simulink model "N3Z_tonetestprevious"  (R2014b)
settings: Solver=ode3  SolverMode=SingleTasking  StartTime=0.0  StopTime=1e-4  FixedStep=fpgaclk  RelTol=1e-3
PreLoadFcn:
  | %fpgaclk=1/32.768e6
  | fpgaclk=1/49.162e6
  | 
  | SerialData=[1,zeros(1,11),1,0,0,1]
  | load ../N3workingG/window
  | win=win';  %Go back to using flatter and wider windowed sync function
  | %load ../N3workingG/hanning    %use Hahn window
  | 
  | load ../N3workingG/PREemphasis   %For pre-empasis and deemphasis FIRs
  | 
  | %LUT3=xls2LUT2('../IQI_Qdemod.xls'); LUT3
  | load ../N3workingG/LUT3
  | load ../N3workingG/FIRiq2
  | % xls2LUT
  | 
  | GetProgFiles
  | 
  | PinAssignments    %Get Pin references for TE0722
  | 
  | 
  | 
  | 
  | 
  | %LCD
  | LCDdata=[LCD_D7,LCD_D6,LCD_D5,LCD_D4,LCD_D3,LCD_D2,LCD_D1,LCD_D0] %Note MSB...LSB!
  | LCDctrl=[LCD_E,LCD_RW,LCD_RS];
  | 
  | %for RS232 on pins 3 and 5 of USBB
  | 
  | %BT chip connections for WT12
  | 
  | RX_BT=RXD
  | TX_BT=TXD
  | 
  | RST_BB=RES
  | 
  | %PCMC=PCMC
  | %PCMS=PCMS
  | %PCMI=PCMI
  | %PCMO=PCMO
  | 
  | %Aliases:
  | SRDBT=PCMI
  | STDBT=PCMO
  | SCLK_BT=PCMC
  | SFS_BT=PCMS
  | 
  | %ADC control
  | 
  | %SDOA=SDOA
  | %SDOB=SDOB
  | %SCK=SCK
  | CONV=Csbar
  | CAL=Cal
  | 
  | ADC_G=[ADC_G3,ADC_G2,ADC_G1,ADC_G0]
  | %PD settings hard coded now
  | 
  | %%%%%%
  | TX_LOW=TX_Low
  | ... (+11 lines)
StartFcn:
  | SerialData=[1,zeros(1,11),1,0,0,1]
values from neighbouring files (symbols this model uses):
  ADC_G0 = {'P10'}    [PinAssignments.m]
  ADC_G1 = {'P11'}    [PinAssignments.m]
  ADC_G2 = {'N14'}    [PinAssignments.m]
  ADC_G3 = {'M11'}    [PinAssignments.m]
  Cal = {'L12'}    [PinAssignments.m]
  Csbar = {'M12'}    [PinAssignments.m]
  LCD_D0 = {'J13'}    [PinAssignments.m]
  LCD_D1 = {'J14'}    [PinAssignments.m]
  LCD_D2 = {'F15'}    [PinAssignments.m]
  LCD_D3 = {'H14'}    [PinAssignments.m]
  LCD_D4 = {'G12'}    [PinAssignments.m]
  LCD_D5 = {'L15'}    [PinAssignments.m]
  LCD_D6 = {'M14'}    [PinAssignments.m]
  LCD_D7 = {'K15'}    [PinAssignments.m]
  PCMC = {'H11'}    [PinAssignments.m]
  PCMI = {'H12'}    [PinAssignments.m]
  PCMO = {'N13'}    [PinAssignments.m]
  PCMS = {'M10'}    [PinAssignments.m]
  RES = {'G11'}    [PinAssignments.m]
  RXD = {'H13'}    [PinAssignments.m]
  TX_Low = {'P15'}    [PinAssignments.m]
  TXD = {'P13'}    [PinAssignments.m]
undefined symbols (not defined in the file or in its folder): AXI4, FIRRX, FIRTX, Lite
libraries: xbsIndex_r4 x1250, MyFunctions x43
(part 9 of 10)

== system N3Z_tonetestprevious/ToneDetect/OutputRegister/Subsystem4 ==
  Data : Inport
  PortId : Inport  Port=2
  Write : Inport  Port=3
  Logical : xbsIndex_r4/Logical  logical_function=AND  inputs=2  en=off  latency=0  precision=Full  arith_type=Unsigned  n_bits=8  bin_pt=2  align_bp=on  dbl_ovrd=off  block_type=logical
      settings: xl_area=[1 0 0 1 0 0 0]  block_version=VER_STRING_GOES_HERE
  PortAddress : xbsIndex_r4/Constant  const=2  gui_display_data_type=Fixed-point  arith_type=Unsigned  n_bits=8  bin_pt=0  preci_type=Single  exp_width=8  frac_width=24  explicit_period=on  period=fpgaclk  equ=P=C  opselect=C  inp2=PCIN>>17  opr=+  inp1=P  carry=CIN  dbl_ovrd=off  block_type=constant
      settings: block_version=VER_STRING_GOES_HERE
  Register1 : xbsIndex_r4/Register  init=0  rst=off  en=on  dbl_ovrd=off  block_type=register
      settings: xl_area=[4 8 0 0 0 0 0]  block_version=VER_STRING_GOES_HERE
  Relational1 : xbsIndex_r4/Relational  mode=a=b  op_type=Bool  en=off  latency=0  dbl_ovrd=off  block_type=relational
      settings: xl_area=[2 0 0 4 0 0 0]  block_version=VER_STRING_GOES_HERE
  LatchedData : Outport
  wires:
  Relational1/1 -> Logical/1
  Logical/1 -> Register1/2
  PortAddress/1 -> Relational1/2
  Data/1 -> Register1/1
  PortId/1 -> Relational1/1
  Write/1 -> Logical/2
  Register1/1 -> LatchedData/1

== system N3Z_tonetestprevious/ToneDetect/OutputRegister/Subsystem5 ==
  Data : Inport
  PortId : Inport  Port=2
  Write : Inport  Port=3
  Logical : xbsIndex_r4/Logical  logical_function=AND  inputs=2  en=off  latency=0  precision=Full  arith_type=Unsigned  n_bits=8  bin_pt=2  align_bp=on  dbl_ovrd=off  block_type=logical
      settings: xl_area=[1 0 0 1 0 0 0]  block_version=VER_STRING_GOES_HERE
  PortAddress : xbsIndex_r4/Constant  const=8  gui_display_data_type=Fixed-point  arith_type=Unsigned  n_bits=8  bin_pt=0  preci_type=Single  exp_width=8  frac_width=24  explicit_period=on  period=fpgaclk  equ=P=C  opselect=C  inp2=PCIN>>17  opr=+  inp1=P  carry=CIN  dbl_ovrd=off  block_type=constant
      settings: block_version=VER_STRING_GOES_HERE
  Register1 : xbsIndex_r4/Register  init=0  rst=off  en=on  dbl_ovrd=off  block_type=register
      settings: xl_area=[4 8 0 0 0 0 0]  block_version=VER_STRING_GOES_HERE
  Relational1 : xbsIndex_r4/Relational  mode=a=b  op_type=Bool  en=off  latency=0  dbl_ovrd=off  block_type=relational
      settings: xl_area=[2 0 0 4 0 0 0]  block_version=VER_STRING_GOES_HERE
  LatchedData : Outport
  Strobe : Outport  Port=2
  wires:
  Relational1/1 -> Logical/1
  Logical/1 -> Register1/2, Strobe/1
  PortAddress/1 -> Relational1/2
  Data/1 -> Register1/1
  PortId/1 -> Relational1/1
  Write/1 -> Logical/2
  Register1/1 -> LatchedData/1

== system N3Z_tonetestprevious/ToneDetect/OutputRegister/Subsystem6 ==
  Data : Inport
  PortId : Inport  Port=2
  Write : Inport  Port=3
  Logical : xbsIndex_r4/Logical  logical_function=AND  inputs=2  en=off  latency=0  precision=Full  arith_type=Unsigned  n_bits=8  bin_pt=2  align_bp=on  dbl_ovrd=off  block_type=logical
      settings: xl_area=[1 0 0 1 0 0 0]  block_version=VER_STRING_GOES_HERE
  PortAddress : xbsIndex_r4/Constant  const=13  gui_display_data_type=Fixed-point  arith_type=Unsigned  n_bits=8  bin_pt=0  preci_type=Single  exp_width=8  frac_width=24  explicit_period=on  period=fpgaclk  equ=P=C  opselect=C  inp2=PCIN>>17  opr=+  inp1=P  carry=CIN  dbl_ovrd=off  block_type=constant
      settings: block_version=VER_STRING_GOES_HERE
  Register1 : xbsIndex_r4/Register  init=0  rst=off  en=on  dbl_ovrd=off  block_type=register
      settings: xl_area=[4 8 0 0 0 0 0]  block_version=VER_STRING_GOES_HERE
  Relational1 : xbsIndex_r4/Relational  mode=a=b  op_type=Bool  en=off  latency=0  dbl_ovrd=off  block_type=relational
      settings: xl_area=[2 0 0 4 0 0 0]  block_version=VER_STRING_GOES_HERE
  LatchedData : Outport
  Strobe : Outport  Port=2
  wires:
  Relational1/1 -> Logical/1
  Logical/1 -> Register1/2, Strobe/1
  PortAddress/1 -> Relational1/2
  Data/1 -> Register1/1
  PortId/1 -> Relational1/1
  Write/1 -> Logical/2
  Register1/1 -> LatchedData/1

== system N3Z_tonetestprevious/ToneDetect/OutputRegister/Subsystem7 ==
  Data : Inport
  PortId : Inport  Port=2
  Write : Inport  Port=3
  Logical : xbsIndex_r4/Logical  logical_function=AND  inputs=2  en=off  latency=0  precision=Full  arith_type=Unsigned  n_bits=8  bin_pt=2  align_bp=on  dbl_ovrd=off  block_type=logical
      settings: xl_area=[1 0 0 1 0 0 0]  block_version=VER_STRING_GOES_HERE
  PortAddress : xbsIndex_r4/Constant  const=18  gui_display_data_type=Fixed-point  arith_type=Unsigned  n_bits=8  bin_pt=0  preci_type=Single  exp_width=8  frac_width=24  explicit_period=on  period=fpgaclk  equ=P=C  opselect=C  inp2=PCIN>>17  opr=+  inp1=P  carry=CIN  dbl_ovrd=off  block_type=constant
      settings: block_version=VER_STRING_GOES_HERE
  Register1 : xbsIndex_r4/Register  init=0  rst=off  en=on  dbl_ovrd=off  block_type=register
      settings: xl_area=[4 8 0 0 0 0 0]  block_version=VER_STRING_GOES_HERE
  Relational1 : xbsIndex_r4/Relational  mode=a=b  op_type=Bool  en=off  latency=0  dbl_ovrd=off  block_type=relational
      settings: xl_area=[2 0 0 4 0 0 0]  block_version=VER_STRING_GOES_HERE
  LatchedData : Outport
  Strobe : Outport  Port=2
  wires:
  Relational1/1 -> Logical/1
  Logical/1 -> Register1/2, Strobe/1
  PortAddress/1 -> Relational1/2
  Data/1 -> Register1/1
  PortId/1 -> Relational1/1
  Write/1 -> Logical/2
  Register1/1 -> LatchedData/1

== system N3Z_tonetestprevious/ToneDetect/OutputRegister/Subsystem8 ==
  Data : Inport
  PortId : Inport  Port=2
  Write : Inport  Port=3
  Logical : xbsIndex_r4/Logical  logical_function=AND  inputs=2  en=off  latency=0  precision=Full  arith_type=Unsigned  n_bits=8  bin_pt=2  align_bp=on  dbl_ovrd=off  block_type=logical
      settings: xl_area=[1 0 0 1 0 0 0]  block_version=VER_STRING_GOES_HERE
  PortAddress : xbsIndex_r4/Constant  const=23  gui_display_data_type=Fixed-point  arith_type=Unsigned  n_bits=8  bin_pt=0  preci_type=Single  exp_width=8  frac_width=24  explicit_period=on  period=fpgaclk  equ=P=C  opselect=C  inp2=PCIN>>17  opr=+  inp1=P  carry=CIN  dbl_ovrd=off  block_type=constant
      settings: block_version=VER_STRING_GOES_HERE
  Register1 : xbsIndex_r4/Register  init=0  rst=off  en=on  dbl_ovrd=off  block_type=register
      settings: xl_area=[4 8 0 0 0 0 0]  block_version=VER_STRING_GOES_HERE
  Relational1 : xbsIndex_r4/Relational  mode=a=b  op_type=Bool  en=off  latency=0  dbl_ovrd=off  block_type=relational
      settings: xl_area=[2 0 0 4 0 0 0]  block_version=VER_STRING_GOES_HERE
  LatchedData : Outport
  Strobe : Outport  Port=2
  wires:
  Relational1/1 -> Logical/1
  Logical/1 -> Register1/2, Strobe/1
  PortAddress/1 -> Relational1/2
  Data/1 -> Register1/1
  PortId/1 -> Relational1/1
  Write/1 -> Logical/2
  Register1/1 -> LatchedData/1

== system N3Z_tonetestprevious/ToneDetect/OutputRegister/Subsystem9 ==
  Data : Inport
  PortId : Inport  Port=2
  Write : Inport  Port=3
  Logical : xbsIndex_r4/Logical  logical_function=AND  inputs=2  en=off  latency=0  precision=Full  arith_type=Unsigned  n_bits=8  bin_pt=2  align_bp=on  dbl_ovrd=off  block_type=logical
      settings: xl_area=[1 0 0 1 0 0 0]  block_version=VER_STRING_GOES_HERE
  PortAddress : xbsIndex_r4/Constant  const=9  gui_display_data_type=Fixed-point  arith_type=Unsigned  n_bits=8  bin_pt=0  preci_type=Single  exp_width=8  frac_width=24  explicit_period=on  period=fpgaclk  equ=P=C  opselect=C  inp2=PCIN>>17  opr=+  inp1=P  carry=CIN  dbl_ovrd=off  block_type=constant
      settings: block_version=VER_STRING_GOES_HERE
  Register1 : xbsIndex_r4/Register  init=0  rst=off  en=on  dbl_ovrd=off  block_type=register
      settings: xl_area=[4 8 0 0 0 0 0]  block_version=VER_STRING_GOES_HERE
  Relational1 : xbsIndex_r4/Relational  mode=a=b  op_type=Bool  en=off  latency=0  dbl_ovrd=off  block_type=relational
      settings: xl_area=[2 0 0 4 0 0 0]  block_version=VER_STRING_GOES_HERE
  LatchedData : Outport
  Strobe : Outport  Port=2
  wires:
  Relational1/1 -> Logical/1
  Logical/1 -> Register1/2, Strobe/1
  PortAddress/1 -> Relational1/2
  Data/1 -> Register1/1
  PortId/1 -> Relational1/1
  Write/1 -> Logical/2
  Register1/1 -> LatchedData/1

== system N3Z_tonetestprevious/User_Interface/OutputRegister/Subsystem ==
  Data : Inport
  PortId : Inport  Port=2
  Write : Inport  Port=3
  Logical : xbsIndex_r4/Logical  logical_function=AND  inputs=2  en=off  latency=0  precision=Full  arith_type=Unsigned  n_bits=8  bin_pt=2  align_bp=on  dbl_ovrd=off  block_type=logical
      settings: xl_area=[1 0 0 1 0 0 0]  block_version=VER_STRING_GOES_HERE
  PortAddress : xbsIndex_r4/Constant  const=0  gui_display_data_type=Fixed-point  arith_type=Unsigned  n_bits=8  bin_pt=0  preci_type=Single  exp_width=8  frac_width=24  explicit_period=on  period=fpgaclk  equ=P=C  opselect=C  inp2=PCIN>>17  opr=+  inp1=P  carry=CIN  dbl_ovrd=off  block_type=constant
      settings: block_version=VER_STRING_GOES_HERE
  Register1 : xbsIndex_r4/Register  init=0  rst=off  en=on  dbl_ovrd=off  block_type=register
      settings: xl_area=[4 8 0 0 0 0 0]  block_version=VER_STRING_GOES_HERE
  Relational1 : xbsIndex_r4/Relational  mode=a=b  op_type=Bool  en=off  latency=0  dbl_ovrd=off  block_type=relational
      settings: xl_area=[2 0 0 4 0 0 0]  block_version=VER_STRING_GOES_HERE
  LatchedData : Outport
  Strobe : Outport  Port=2
  wires:
  Relational1/1 -> Logical/1
  Logical/1 -> Register1/2, Strobe/1
  PortAddress/1 -> Relational1/2
  Data/1 -> Register1/1
  PortId/1 -> Relational1/1
  Write/1 -> Logical/2
  Register1/1 -> LatchedData/1

== system N3Z_tonetestprevious/User_Interface/OutputRegister/Subsystem1 ==
  Data : Inport
  PortId : Inport  Port=2
  Write : Inport  Port=3
  Logical : xbsIndex_r4/Logical  logical_function=AND  inputs=2  en=off  latency=0  precision=Full  arith_type=Unsigned  n_bits=8  bin_pt=2  align_bp=on  dbl_ovrd=off  block_type=logical
      settings: xl_area=[1 0 0 1 0 0 0]  block_version=VER_STRING_GOES_HERE
  PortAddress : xbsIndex_r4/Constant  const=1  gui_display_data_type=Fixed-point  arith_type=Unsigned  n_bits=8  bin_pt=0  preci_type=Single  exp_width=8  frac_width=24  explicit_period=on  period=fpgaclk  equ=P=C  opselect=C  inp2=PCIN>>17  opr=+  inp1=P  carry=CIN  dbl_ovrd=off  block_type=constant
      settings: block_version=VER_STRING_GOES_HERE
  Register1 : xbsIndex_r4/Register  init=0  rst=off  en=on  dbl_ovrd=off  block_type=register
      settings: xl_area=[4 8 0 0 0 0 0]  block_version=VER_STRING_GOES_HERE
  Register2 : xbsIndex_r4/Register  init=0  rst=off  en=off  dbl_ovrd=off  block_type=register
      settings: xl_area=[1 1 0 0 0 0 0]  block_version=VER_STRING_GOES_HERE
  Register3 : xbsIndex_r4/Register  init=0  rst=off  en=off  dbl_ovrd=off  block_type=register
      settings: xl_area=[1 1 0 0 0 0 0]  block_version=VER_STRING_GOES_HERE
  Relational1 : xbsIndex_r4/Relational  mode=a=b  op_type=Bool  en=off  latency=0  dbl_ovrd=off  block_type=relational
      settings: xl_area=[2 0 0 4 0 0 0]  block_version=VER_STRING_GOES_HERE
  pulse2 : Subsystem
  LatchedData : Outport
  MemWrite : Outport  Port=2
  wires:
  Relational1/1 -> Logical/1
  Logical/1 -> Register1/2, Register3/1
  PortAddress/1 -> Relational1/2
  Data/1 -> Register1/1
  PortId/1 -> Relational1/1
  Write/1 -> Logical/2
  Register1/1 -> LatchedData/1
  Register2/1 -> pulse2/1(In1)
  Register3/1 -> Register2/1
  pulse2/1(Out1) -> MemWrite/1

== system N3Z_tonetestprevious/User_Interface/OutputRegister/Subsystem10 ==
  Data : Inport
  PortId : Inport  Port=2
  Write : Inport  Port=3
  Logical : xbsIndex_r4/Logical  logical_function=AND  inputs=2  en=off  latency=0  precision=Full  arith_type=Unsigned  n_bits=8  bin_pt=2  align_bp=on  dbl_ovrd=off  block_type=logical
      settings: xl_area=[1 0 0 1 0 0 0]  block_version=VER_STRING_GOES_HERE
  PortAddress : xbsIndex_r4/Constant  const=10  gui_display_data_type=Fixed-point  arith_type=Unsigned  n_bits=8  bin_pt=0  preci_type=Single  exp_width=8  frac_width=24  explicit_period=on  period=fpgaclk  equ=P=C  opselect=C  inp2=PCIN>>17  opr=+  inp1=P  carry=CIN  dbl_ovrd=off  block_type=constant
      settings: block_version=VER_STRING_GOES_HERE
  Register1 : xbsIndex_r4/Register  init=floor(30022/256)  rst=off  en=on  dbl_ovrd=off  block_type=register
      settings: xl_area=[4 8 0 0 0 0 0]  block_version=VER_STRING_GOES_HERE
  Relational1 : xbsIndex_r4/Relational  mode=a=b  op_type=Bool  en=off  latency=0  dbl_ovrd=off  block_type=relational
      settings: xl_area=[2 0 0 4 0 0 0]  block_version=VER_STRING_GOES_HERE
  LatchedData : Outport
  wires:
  Relational1/1 -> Logical/1
  Logical/1 -> Register1/2
  PortAddress/1 -> Relational1/2
  Data/1 -> Register1/1
  PortId/1 -> Relational1/1
  Write/1 -> Logical/2
  Register1/1 -> LatchedData/1

== system N3Z_tonetestprevious/User_Interface/OutputRegister/Subsystem11 ==
  Data : Inport
  PortId : Inport  Port=2
  Write : Inport  Port=3
  Logical : xbsIndex_r4/Logical  logical_function=AND  inputs=2  en=off  latency=0  precision=Full  arith_type=Unsigned  n_bits=8  bin_pt=2  align_bp=on  dbl_ovrd=off  block_type=logical
      settings: xl_area=[1 0 0 1 0 0 0]  block_version=VER_STRING_GOES_HERE
  PortAddress : xbsIndex_r4/Constant  const=11  gui_display_data_type=Fixed-point  arith_type=Unsigned  n_bits=8  bin_pt=0  preci_type=Single  exp_width=8  frac_width=24  explicit_period=on  period=fpgaclk  equ=P=C  opselect=C  inp2=PCIN>>17  opr=+  inp1=P  carry=CIN  dbl_ovrd=off  block_type=constant
      settings: block_version=VER_STRING_GOES_HERE
  Register1 : xbsIndex_r4/Register  init=mod(30022 ,256)  rst=off  en=on  dbl_ovrd=off  block_type=register
      settings: xl_area=[4 8 0 0 0 0 0]  block_version=VER_STRING_GOES_HERE
  Relational1 : xbsIndex_r4/Relational  mode=a=b  op_type=Bool  en=off  latency=0  dbl_ovrd=off  block_type=relational
      settings: xl_area=[2 0 0 4 0 0 0]  block_version=VER_STRING_GOES_HERE
  LatchedData : Outport
  wires:
  Relational1/1 -> Logical/1
  Logical/1 -> Register1/2
  PortAddress/1 -> Relational1/2
  Data/1 -> Register1/1
  PortId/1 -> Relational1/1
  Write/1 -> Logical/2
  Register1/1 -> LatchedData/1

== system N3Z_tonetestprevious/User_Interface/OutputRegister/Subsystem12 ==
  note: Set to 149 for about 0.9V to TDA7052A
      | 141 for 0.85V
  Data : Inport
  PortId : Inport  Port=2
  Write : Inport  Port=3
  Logical : xbsIndex_r4/Logical  logical_function=AND  inputs=2  en=off  latency=0  precision=Full  arith_type=Unsigned  n_bits=8  bin_pt=2  align_bp=on  dbl_ovrd=off  block_type=logical
      settings: xl_area=[1 0 0 1 0 0 0]  block_version=VER_STRING_GOES_HERE
  PortAddress : xbsIndex_r4/Constant  const=12  gui_display_data_type=Fixed-point  arith_type=Unsigned  n_bits=8  bin_pt=0  preci_type=Single  exp_width=8  frac_width=24  explicit_period=on  period=fpgaclk  equ=P=C  opselect=C  inp2=PCIN>>17  opr=+  inp1=P  carry=CIN  dbl_ovrd=off  block_type=constant
      settings: block_version=VER_STRING_GOES_HERE
  Register1 : xbsIndex_r4/Register  init=141  rst=off  en=on  dbl_ovrd=off  block_type=register
      settings: xl_area=[4 8 0 0 0 0 0]  block_version=VER_STRING_GOES_HERE
  Relational1 : xbsIndex_r4/Relational  mode=a=b  op_type=Bool  en=off  latency=0  dbl_ovrd=off  block_type=relational
      settings: xl_area=[2 0 0 4 0 0 0]  block_version=VER_STRING_GOES_HERE
  LatchedData : Outport
  wires:
  Relational1/1 -> Logical/1
  Logical/1 -> Register1/2
  PortAddress/1 -> Relational1/2
  Data/1 -> Register1/1
  PortId/1 -> Relational1/1
  Write/1 -> Logical/2
  Register1/1 -> LatchedData/1

== system N3Z_tonetestprevious/User_Interface/OutputRegister/Subsystem13 ==
  Data : Inport
  PortId : Inport  Port=2
  Write : Inport  Port=3
  Logical : xbsIndex_r4/Logical  logical_function=AND  inputs=2  en=off  latency=0  precision=Full  arith_type=Unsigned  n_bits=8  bin_pt=2  align_bp=on  dbl_ovrd=off  block_type=logical
      settings: xl_area=[1 0 0 1 0 0 0]  block_version=VER_STRING_GOES_HERE
  PortAddress : xbsIndex_r4/Constant  const=13  gui_display_data_type=Fixed-point  arith_type=Unsigned  n_bits=8  bin_pt=0  preci_type=Single  exp_width=8  frac_width=24  explicit_period=on  period=fpgaclk  equ=P=C  opselect=C  inp2=PCIN>>17  opr=+  inp1=P  carry=CIN  dbl_ovrd=off  block_type=constant
      settings: block_version=VER_STRING_GOES_HERE
  Register1 : xbsIndex_r4/Register  init=0  rst=off  en=on  dbl_ovrd=off  block_type=register
      settings: xl_area=[4 8 0 0 0 0 0]  block_version=VER_STRING_GOES_HERE
  Relational1 : xbsIndex_r4/Relational  mode=a=b  op_type=Bool  en=off  latency=0  dbl_ovrd=off  block_type=relational
      settings: xl_area=[2 0 0 4 0 0 0]  block_version=VER_STRING_GOES_HERE
  LatchedData : Outport
  wires:
  Relational1/1 -> Logical/1
  Logical/1 -> Register1/2
  PortAddress/1 -> Relational1/2
  Data/1 -> Register1/1
  PortId/1 -> Relational1/1
  Write/1 -> Logical/2
  Register1/1 -> LatchedData/1

== system N3Z_tonetestprevious/User_Interface/OutputRegister/Subsystem14 ==
  Data : Inport
  PortId : Inport  Port=2
  Write : Inport  Port=3
  Logical : xbsIndex_r4/Logical  logical_function=AND  inputs=2  en=off  latency=0  precision=Full  arith_type=Unsigned  n_bits=8  bin_pt=2  align_bp=on  dbl_ovrd=off  block_type=logical
      settings: xl_area=[1 0 0 1 0 0 0]  block_version=VER_STRING_GOES_HERE
  PortAddress : xbsIndex_r4/Constant  const=14  gui_display_data_type=Fixed-point  arith_type=Unsigned  n_bits=8  bin_pt=0  preci_type=Single  exp_width=8  frac_width=24  explicit_period=on  period=fpgaclk  equ=P=C  opselect=C  inp2=PCIN>>17  opr=+  inp1=P  carry=CIN  dbl_ovrd=off  block_type=constant
      settings: block_version=VER_STRING_GOES_HERE
  Register1 : xbsIndex_r4/Register  init=floor(29700/256)  rst=off  en=on  dbl_ovrd=off  block_type=register
      settings: xl_area=[4 8 0 0 0 0 0]  block_version=VER_STRING_GOES_HERE
  Relational1 : xbsIndex_r4/Relational  mode=a=b  op_type=Bool  en=off  latency=0  dbl_ovrd=off  block_type=relational
      settings: xl_area=[2 0 0 4 0 0 0]  block_version=VER_STRING_GOES_HERE
  LatchedData : Outport
  AckFifo : Outport  Port=2
  wires:
  Relational1/1 -> Logical/1
  Logical/1 -> Register1/2, AckFifo/1
  PortAddress/1 -> Relational1/2
  Data/1 -> Register1/1
  PortId/1 -> Relational1/1
  Write/1 -> Logical/2
  Register1/1 -> LatchedData/1

== system N3Z_tonetestprevious/User_Interface/OutputRegister/Subsystem15 ==
  Data : Inport
  PortId : Inport  Port=2
  Write : Inport  Port=3
  Logical : xbsIndex_r4/Logical  logical_function=AND  inputs=2  en=off  latency=0  precision=Full  arith_type=Unsigned  n_bits=8  bin_pt=2  align_bp=on  dbl_ovrd=off  block_type=logical
      settings: xl_area=[1 0 0 1 0 0 0]  block_version=VER_STRING_GOES_HERE
  PortAddress : xbsIndex_r4/Constant  const=22  gui_display_data_type=Fixed-point  arith_type=Unsigned  n_bits=8  bin_pt=0  preci_type=Single  exp_width=8  frac_width=24  explicit_period=on  period=fpgaclk  equ=P=C  opselect=C  inp2=PCIN>>17  opr=+  inp1=P  carry=CIN  dbl_ovrd=off  block_type=constant
      settings: block_version=VER_STRING_GOES_HERE
  Register1 : xbsIndex_r4/Register  init=0  rst=off  en=on  dbl_ovrd=off  block_type=register
      settings: xl_area=[4 8 0 0 0 0 0]  block_version=VER_STRING_GOES_HERE
  Relational1 : xbsIndex_r4/Relational  mode=a=b  op_type=Bool  en=off  latency=0  dbl_ovrd=off  block_type=relational
      settings: xl_area=[2 0 0 4 0 0 0]  block_version=VER_STRING_GOES_HERE
  LatchedData : Outport
  Strobe : Outport  Port=2
  wires:
  Relational1/1 -> Logical/1
  Logical/1 -> Register1/2, Strobe/1
  PortAddress/1 -> Relational1/2
  Data/1 -> Register1/1
  PortId/1 -> Relational1/1
  Write/1 -> Logical/2
  Register1/1 -> LatchedData/1

== system N3Z_tonetestprevious/User_Interface/OutputRegister/Subsystem16 ==
  Data : Inport
  PortId : Inport  Port=2
  Write : Inport  Port=3
  Logical : xbsIndex_r4/Logical  logical_function=AND  inputs=2  en=off  latency=0  precision=Full  arith_type=Unsigned  n_bits=8  bin_pt=2  align_bp=on  dbl_ovrd=off  block_type=logical
      settings: xl_area=[1 0 0 1 0 0 0]  block_version=VER_STRING_GOES_HERE
  PortAddress : xbsIndex_r4/Constant  const=23  gui_display_data_type=Fixed-point  arith_type=Unsigned  n_bits=8  bin_pt=0  preci_type=Single  exp_width=8  frac_width=24  explicit_period=on  period=fpgaclk  equ=P=C  opselect=C  inp2=PCIN>>17  opr=+  inp1=P  carry=CIN  dbl_ovrd=off  block_type=constant
      settings: block_version=VER_STRING_GOES_HERE
  Register1 : xbsIndex_r4/Register  init=0  rst=off  en=on  dbl_ovrd=off  block_type=register
      settings: xl_area=[4 8 0 0 0 0 0]  block_version=VER_STRING_GOES_HERE
  Relational1 : xbsIndex_r4/Relational  mode=a=b  op_type=Bool  en=off  latency=0  dbl_ovrd=off  block_type=relational
      settings: xl_area=[2 0 0 4 0 0 0]  block_version=VER_STRING_GOES_HERE
  LatchedData : Outport
  Strobe : Outport  Port=2
  wires:
  Relational1/1 -> Logical/1
  Logical/1 -> Register1/2, Strobe/1
  PortAddress/1 -> Relational1/2
  Data/1 -> Register1/1
  PortId/1 -> Relational1/1
  Write/1 -> Logical/2
  Register1/1 -> LatchedData/1

== system N3Z_tonetestprevious/User_Interface/OutputRegister/Subsystem17 ==
  Data : Inport
  PortId : Inport  Port=2
  Write : Inport  Port=3
  Logical : xbsIndex_r4/Logical  logical_function=AND  inputs=2  en=off  latency=0  precision=Full  arith_type=Unsigned  n_bits=8  bin_pt=2  align_bp=on  dbl_ovrd=off  block_type=logical
      settings: xl_area=[1 0 0 1 0 0 0]  block_version=VER_STRING_GOES_HERE
  PortAddress : xbsIndex_r4/Constant  const=17  gui_display_data_type=Fixed-point  arith_type=Unsigned  n_bits=8  bin_pt=0  preci_type=Single  exp_width=8  frac_width=24  explicit_period=on  period=fpgaclk  equ=P=C  opselect=C  inp2=PCIN>>17  opr=+  inp1=P  carry=CIN  dbl_ovrd=off  block_type=constant
      settings: block_version=VER_STRING_GOES_HERE
  Register1 : xbsIndex_r4/Register  init=mod(29700,256)  rst=off  en=on  dbl_ovrd=off  block_type=register
      settings: xl_area=[4 8 0 0 0 0 0]  block_version=VER_STRING_GOES_HERE
  Relational1 : xbsIndex_r4/Relational  mode=a=b  op_type=Bool  en=off  latency=0  dbl_ovrd=off  block_type=relational
      settings: xl_area=[2 0 0 4 0 0 0]  block_version=VER_STRING_GOES_HERE
  LatchedData : Outport
  Strobe : Outport  Port=2
  wires:
  Relational1/1 -> Logical/1
  Logical/1 -> Register1/2, Strobe/1
  PortAddress/1 -> Relational1/2
  Data/1 -> Register1/1
  PortId/1 -> Relational1/1
  Write/1 -> Logical/2
  Register1/1 -> LatchedData/1

== system N3Z_tonetestprevious/User_Interface/OutputRegister/Subsystem18 ==
  Data : Inport
  PortId : Inport  Port=2
  Write : Inport  Port=3
  Logical : xbsIndex_r4/Logical  logical_function=AND  inputs=2  en=off  latency=0  precision=Full  arith_type=Unsigned  n_bits=8  bin_pt=2  align_bp=on  dbl_ovrd=off  block_type=logical
      settings: xl_area=[1 0 0 1 0 0 0]  block_version=VER_STRING_GOES_HERE
  PortAddress : xbsIndex_r4/Constant  const=18  gui_display_data_type=Fixed-point  arith_type=Unsigned  n_bits=8  bin_pt=0  preci_type=Single  exp_width=8  frac_width=24  explicit_period=on  period=fpgaclk  equ=P=C  opselect=C  inp2=PCIN>>17  opr=+  inp1=P  carry=CIN  dbl_ovrd=off  block_type=constant
      settings: block_version=VER_STRING_GOES_HERE
  Register1 : xbsIndex_r4/Register  init=mod(29700,256)  rst=off  en=on  dbl_ovrd=off  block_type=register
      settings: xl_area=[4 8 0 0 0 0 0]  block_version=VER_STRING_GOES_HERE
  Relational1 : xbsIndex_r4/Relational  mode=a=b  op_type=Bool  en=off  latency=0  dbl_ovrd=off  block_type=relational
      settings: xl_area=[2 0 0 4 0 0 0]  block_version=VER_STRING_GOES_HERE
  LatchedData : Outport
  Strobe : Outport  Port=2
  wires:
  Relational1/1 -> Logical/1
  Logical/1 -> Register1/2, Strobe/1
  PortAddress/1 -> Relational1/2
  Data/1 -> Register1/1
  PortId/1 -> Relational1/1
  Write/1 -> Logical/2
  Register1/1 -> LatchedData/1

== system N3Z_tonetestprevious/User_Interface/OutputRegister/Subsystem19 ==
  Data : Inport
  PortId : Inport  Port=2
  Write : Inport  Port=3
  Logical : xbsIndex_r4/Logical  logical_function=AND  inputs=2  en=off  latency=0  precision=Full  arith_type=Unsigned  n_bits=8  bin_pt=2  align_bp=on  dbl_ovrd=off  block_type=logical
      settings: xl_area=[1 0 0 1 0 0 0]  block_version=VER_STRING_GOES_HERE
  PortAddress : xbsIndex_r4/Constant  const=19  gui_display_data_type=Fixed-point  arith_type=Unsigned  n_bits=8  bin_pt=0  preci_type=Single  exp_width=8  frac_width=24  explicit_period=on  period=fpgaclk  equ=P=C  opselect=C  inp2=PCIN>>17  opr=+  inp1=P  carry=CIN  dbl_ovrd=off  block_type=constant
      settings: block_version=VER_STRING_GOES_HERE
  Register1 : xbsIndex_r4/Register  init=32  rst=off  en=on  dbl_ovrd=off  block_type=register
      settings: xl_area=[4 8 0 0 0 0 0]  block_version=VER_STRING_GOES_HERE
  Relational1 : xbsIndex_r4/Relational  mode=a=b  op_type=Bool  en=off  latency=0  dbl_ovrd=off  block_type=relational
      settings: xl_area=[2 0 0 4 0 0 0]  block_version=VER_STRING_GOES_HERE
  LatchedData : Outport
  Strobe : Outport  Port=2
  wires:
  Relational1/1 -> Logical/1
  Logical/1 -> Register1/2, Strobe/1
  PortAddress/1 -> Relational1/2
  Data/1 -> Register1/1
  PortId/1 -> Relational1/1
  Write/1 -> Logical/2
  Register1/1 -> LatchedData/1

== system N3Z_tonetestprevious/User_Interface/OutputRegister/Subsystem2 ==
  Data : Inport
  PortId : Inport  Port=2
  Write : Inport  Port=3
  Logical : xbsIndex_r4/Logical  logical_function=AND  inputs=2  en=off  latency=0  precision=Full  arith_type=Unsigned  n_bits=8  bin_pt=2  align_bp=on  dbl_ovrd=off  block_type=logical
      settings: xl_area=[1 0 0 1 0 0 0]  block_version=VER_STRING_GOES_HERE
  PortAddress : xbsIndex_r4/Constant  const=3  gui_display_data_type=Fixed-point  arith_type=Unsigned  n_bits=8  bin_pt=0  preci_type=Single  exp_width=8  frac_width=24  explicit_period=on  period=fpgaclk  equ=P=C  opselect=C  inp2=PCIN>>17  opr=+  inp1=P  carry=CIN  dbl_ovrd=off  block_type=constant
      settings: block_version=VER_STRING_GOES_HERE
  Register1 : xbsIndex_r4/Register  init=0  rst=off  en=on  dbl_ovrd=off  block_type=register
      settings: xl_area=[4 8 0 0 0 0 0]  block_version=VER_STRING_GOES_HERE
  Relational1 : xbsIndex_r4/Relational  mode=a=b  op_type=Bool  en=off  latency=0  dbl_ovrd=off  block_type=relational
      settings: xl_area=[2 0 0 4 0 0 0]  block_version=VER_STRING_GOES_HERE
  LatchedData : Outport
  wires:
  Relational1/1 -> Logical/1
  Logical/1 -> Register1/2
  PortAddress/1 -> Relational1/2
  Data/1 -> Register1/1
  PortId/1 -> Relational1/1
  Write/1 -> Logical/2
  Register1/1 -> LatchedData/1

== system N3Z_tonetestprevious/User_Interface/OutputRegister/Subsystem20 ==
  Data : Inport
  PortId : Inport  Port=2
  Write : Inport  Port=3
  Logical : xbsIndex_r4/Logical  logical_function=AND  inputs=2  en=off  latency=0  precision=Full  arith_type=Unsigned  n_bits=8  bin_pt=2  align_bp=on  dbl_ovrd=off  block_type=logical
      settings: xl_area=[1 0 0 1 0 0 0]  block_version=VER_STRING_GOES_HERE
  PortAddress : xbsIndex_r4/Constant  const=20  gui_display_data_type=Fixed-point  arith_type=Unsigned  n_bits=8  bin_pt=0  preci_type=Single  exp_width=8  frac_width=24  explicit_period=on  period=fpgaclk  equ=P=C  opselect=C  inp2=PCIN>>17  opr=+  inp1=P  carry=CIN  dbl_ovrd=off  block_type=constant
      settings: block_version=VER_STRING_GOES_HERE
  Register1 : xbsIndex_r4/Register  init=0  rst=off  en=on  dbl_ovrd=off  block_type=register
      settings: xl_area=[4 8 0 0 0 0 0]  block_version=VER_STRING_GOES_HERE
  Relational1 : xbsIndex_r4/Relational  mode=a=b  op_type=Bool  en=off  latency=0  dbl_ovrd=off  block_type=relational
      settings: xl_area=[2 0 0 4 0 0 0]  block_version=VER_STRING_GOES_HERE
  LatchedData : Outport
  Strobe : Outport  Port=2
  wires:
  Relational1/1 -> Logical/1
  Logical/1 -> Register1/2, Strobe/1
  PortAddress/1 -> Relational1/2
  Data/1 -> Register1/1
  PortId/1 -> Relational1/1
  Write/1 -> Logical/2
  Register1/1 -> LatchedData/1

== system N3Z_tonetestprevious/User_Interface/OutputRegister/Subsystem21 ==
  Data : Inport
  PortId : Inport  Port=2
  Write : Inport  Port=3
  Logical : xbsIndex_r4/Logical  logical_function=AND  inputs=2  en=off  latency=0  precision=Full  arith_type=Unsigned  n_bits=8  bin_pt=2  align_bp=on  dbl_ovrd=off  block_type=logical
      settings: xl_area=[1 0 0 1 0 0 0]  block_version=VER_STRING_GOES_HERE
  PortAddress : xbsIndex_r4/Constant  const=21  gui_display_data_type=Fixed-point  arith_type=Unsigned  n_bits=8  bin_pt=0  preci_type=Single  exp_width=8  frac_width=24  explicit_period=on  period=fpgaclk  equ=P=C  opselect=C  inp2=PCIN>>17  opr=+  inp1=P  carry=CIN  dbl_ovrd=off  block_type=constant
      settings: block_version=VER_STRING_GOES_HERE
  Register1 : xbsIndex_r4/Register  init=0  rst=off  en=on  dbl_ovrd=off  block_type=register
      settings: xl_area=[4 8 0 0 0 0 0]  block_version=VER_STRING_GOES_HERE
  Relational1 : xbsIndex_r4/Relational  mode=a=b  op_type=Bool  en=off  latency=0  dbl_ovrd=off  block_type=relational
      settings: xl_area=[2 0 0 4 0 0 0]  block_version=VER_STRING_GOES_HERE
  LatchedData : Outport
  Strobe : Outport  Port=2
  wires:
  Relational1/1 -> Logical/1
  Logical/1 -> Register1/2, Strobe/1
  PortAddress/1 -> Relational1/2
  Data/1 -> Register1/1
  PortId/1 -> Relational1/1
  Write/1 -> Logical/2
  Register1/1 -> LatchedData/1

== system N3Z_tonetestprevious/User_Interface/OutputRegister/Subsystem22 ==
  Data : Inport
  PortId : Inport  Port=2
  Write : Inport  Port=3
  Logical : xbsIndex_r4/Logical  logical_function=AND  inputs=2  en=off  latency=0  precision=Full  arith_type=Unsigned  n_bits=8  bin_pt=2  align_bp=on  dbl_ovrd=off  block_type=logical
      settings: xl_area=[1 0 0 1 0 0 0]  block_version=VER_STRING_GOES_HERE
  PortAddress : xbsIndex_r4/Constant  const=24  gui_display_data_type=Fixed-point  arith_type=Unsigned  n_bits=8  bin_pt=0  preci_type=Single  exp_width=8  frac_width=24  explicit_period=on  period=fpgaclk  equ=P=C  opselect=C  inp2=PCIN>>17  opr=+  inp1=P  carry=CIN  dbl_ovrd=off  block_type=constant
      settings: block_version=VER_STRING_GOES_HERE
  Register1 : xbsIndex_r4/Register  init=0  rst=off  en=on  dbl_ovrd=off  block_type=register
      settings: xl_area=[4 8 0 0 0 0 0]  block_version=VER_STRING_GOES_HERE
  Relational1 : xbsIndex_r4/Relational  mode=a=b  op_type=Bool  en=off  latency=0  dbl_ovrd=off  block_type=relational
      settings: xl_area=[2 0 0 4 0 0 0]  block_version=VER_STRING_GOES_HERE
  LatchedData : Outport
  Strobe : Outport  Port=2
  wires:
  Relational1/1 -> Logical/1
  Logical/1 -> Register1/2, Strobe/1
  PortAddress/1 -> Relational1/2
  Data/1 -> Register1/1
  PortId/1 -> Relational1/1
  Write/1 -> Logical/2
  Register1/1 -> LatchedData/1

== system N3Z_tonetestprevious/User_Interface/OutputRegister/Subsystem23 ==
  Data : Inport
  PortId : Inport  Port=2
  Write : Inport  Port=3
  Logical : xbsIndex_r4/Logical  logical_function=AND  inputs=2  en=off  latency=0  precision=Full  arith_type=Unsigned  n_bits=8  bin_pt=2  align_bp=on  dbl_ovrd=off  block_type=logical
      settings: xl_area=[1 0 0 1 0 0 0]  block_version=VER_STRING_GOES_HERE
  PortAddress : xbsIndex_r4/Constant  const=25  gui_display_data_type=Fixed-point  arith_type=Unsigned  n_bits=8  bin_pt=0  preci_type=Single  exp_width=8  frac_width=24  explicit_period=on  period=fpgaclk  equ=P=C  opselect=C  inp2=PCIN>>17  opr=+  inp1=P  carry=CIN  dbl_ovrd=off  block_type=constant
      settings: block_version=VER_STRING_GOES_HERE
  Register1 : xbsIndex_r4/Register  init=0  rst=off  en=on  dbl_ovrd=off  block_type=register
      settings: xl_area=[4 8 0 0 0 0 0]  block_version=VER_STRING_GOES_HERE
  Relational1 : xbsIndex_r4/Relational  mode=a=b  op_type=Bool  en=off  latency=0  dbl_ovrd=off  block_type=relational
      settings: xl_area=[2 0 0 4 0 0 0]  block_version=VER_STRING_GOES_HERE
  LatchedData : Outport
  Strobe : Outport  Port=2
  wires:
  Relational1/1 -> Logical/1
  Logical/1 -> Register1/2, Strobe/1
  PortAddress/1 -> Relational1/2
  Data/1 -> Register1/1
  PortId/1 -> Relational1/1
  Write/1 -> Logical/2
  Register1/1 -> LatchedData/1

== system N3Z_tonetestprevious/User_Interface/OutputRegister/Subsystem3 ==
  Data : Inport
  PortId : Inport  Port=2
  Write : Inport  Port=3
  Logical : xbsIndex_r4/Logical  logical_function=AND  inputs=2  en=off  latency=0  precision=Full  arith_type=Unsigned  n_bits=8  bin_pt=2  align_bp=on  dbl_ovrd=off  block_type=logical
      settings: xl_area=[1 0 0 1 0 0 0]  block_version=VER_STRING_GOES_HERE
  PortAddress : xbsIndex_r4/Constant  const=4  gui_display_data_type=Fixed-point  arith_type=Unsigned  n_bits=8  bin_pt=0  preci_type=Single  exp_width=8  frac_width=24  explicit_period=on  period=fpgaclk  equ=P=C  opselect=C  inp2=PCIN>>17  opr=+  inp1=P  carry=CIN  dbl_ovrd=off  block_type=constant
      settings: block_version=VER_STRING_GOES_HERE
  Register1 : xbsIndex_r4/Register  init=0  rst=off  en=on  dbl_ovrd=off  block_type=register
      settings: xl_area=[4 8 0 0 0 0 0]  block_version=VER_STRING_GOES_HERE
  Relational1 : xbsIndex_r4/Relational  mode=a=b  op_type=Bool  en=off  latency=0  dbl_ovrd=off  block_type=relational
      settings: xl_area=[2 0 0 4 0 0 0]  block_version=VER_STRING_GOES_HERE
  LatchedData : Outport
  wires:
  Relational1/1 -> Logical/1
  Logical/1 -> Register1/2
  PortAddress/1 -> Relational1/2
  Data/1 -> Register1/1
  PortId/1 -> Relational1/1
  Write/1 -> Logical/2
  Register1/1 -> LatchedData/1

== system N3Z_tonetestprevious/User_Interface/OutputRegister/Subsystem4 ==
  Data : Inport
  PortId : Inport  Port=2
  Write : Inport  Port=3
  Logical : xbsIndex_r4/Logical  logical_function=AND  inputs=2  en=off  latency=0  precision=Full  arith_type=Unsigned  n_bits=8  bin_pt=2  align_bp=on  dbl_ovrd=off  block_type=logical
      settings: xl_area=[1 0 0 1 0 0 0]  block_version=VER_STRING_GOES_HERE
  PortAddress : xbsIndex_r4/Constant  const=5  gui_display_data_type=Fixed-point  arith_type=Unsigned  n_bits=8  bin_pt=0  preci_type=Single  exp_width=8  frac_width=24  explicit_period=on  period=fpgaclk  equ=P=C  opselect=C  inp2=PCIN>>17  opr=+  inp1=P  carry=CIN  dbl_ovrd=off  block_type=constant
      settings: block_version=VER_STRING_GOES_HERE
  Register1 : xbsIndex_r4/Register  init=0  rst=off  en=on  dbl_ovrd=off  block_type=register
      settings: xl_area=[4 8 0 0 0 0 0]  block_version=VER_STRING_GOES_HERE
  Relational1 : xbsIndex_r4/Relational  mode=a=b  op_type=Bool  en=off  latency=0  dbl_ovrd=off  block_type=relational
      settings: xl_area=[2 0 0 4 0 0 0]  block_version=VER_STRING_GOES_HERE
  LatchedData : Outport
  wires:
  Relational1/1 -> Logical/1
  Logical/1 -> Register1/2
  PortAddress/1 -> Relational1/2
  Data/1 -> Register1/1
  PortId/1 -> Relational1/1
  Write/1 -> Logical/2
  Register1/1 -> LatchedData/1

== system N3Z_tonetestprevious/User_Interface/OutputRegister/Subsystem5 ==
  Data : Inport
  PortId : Inport  Port=2
  Write : Inport  Port=3
  Logical : xbsIndex_r4/Logical  logical_function=AND  inputs=2  en=off  latency=0  precision=Full  arith_type=Unsigned  n_bits=8  bin_pt=2  align_bp=on  dbl_ovrd=off  block_type=logical
      settings: xl_area=[1 0 0 1 0 0 0]  block_version=VER_STRING_GOES_HERE
  PortAddress : xbsIndex_r4/Constant  const=6  gui_display_data_type=Fixed-point  arith_type=Unsigned  n_bits=8  bin_pt=0  preci_type=Single  exp_width=8  frac_width=24  explicit_period=on  period=fpgaclk  equ=P=C  opselect=C  inp2=PCIN>>17  opr=+  inp1=P  carry=CIN  dbl_ovrd=off  block_type=constant
      settings: block_version=VER_STRING_GOES_HERE
  Register1 : xbsIndex_r4/Register  init=0  rst=off  en=on  dbl_ovrd=off  block_type=register
      settings: xl_area=[4 8 0 0 0 0 0]  block_version=VER_STRING_GOES_HERE
  Relational1 : xbsIndex_r4/Relational  mode=a=b  op_type=Bool  en=off  latency=0  dbl_ovrd=off  block_type=relational
      settings: xl_area=[2 0 0 4 0 0 0]  block_version=VER_STRING_GOES_HERE
  LatchedData : Outport
  wires:
  Relational1/1 -> Logical/1
  Logical/1 -> Register1/2
  PortAddress/1 -> Relational1/2
  Data/1 -> Register1/1
  PortId/1 -> Relational1/1
  Write/1 -> Logical/2
  Register1/1 -> LatchedData/1

== system N3Z_tonetestprevious/User_Interface/OutputRegister/Subsystem6 ==
  Data : Inport
  PortId : Inport  Port=2
  Write : Inport  Port=3
  Logical : xbsIndex_r4/Logical  logical_function=AND  inputs=2  en=off  latency=0  precision=Full  arith_type=Unsigned  n_bits=8  bin_pt=2  align_bp=on  dbl_ovrd=off  block_type=logical
      settings: xl_area=[1 0 0 1 0 0 0]  block_version=VER_STRING_GOES_HERE
  PortAddress : xbsIndex_r4/Constant  const=7  gui_display_data_type=Fixed-point  arith_type=Unsigned  n_bits=8  bin_pt=0  preci_type=Single  exp_width=8  frac_width=24  explicit_period=on  period=fpgaclk  equ=P=C  opselect=C  inp2=PCIN>>17  opr=+  inp1=P  carry=CIN  dbl_ovrd=off  block_type=constant
      settings: block_version=VER_STRING_GOES_HERE
  Register1 : xbsIndex_r4/Register  init=0  rst=off  en=on  dbl_ovrd=off  block_type=register
      settings: xl_area=[4 8 0 0 0 0 0]  block_version=VER_STRING_GOES_HERE
  Relational1 : xbsIndex_r4/Relational  mode=a=b  op_type=Bool  en=off  latency=0  dbl_ovrd=off  block_type=relational
      settings: xl_area=[2 0 0 4 0 0 0]  block_version=VER_STRING_GOES_HERE
  LatchedData : Outport
  wires:
  Relational1/1 -> Logical/1
  Logical/1 -> Register1/2
  PortAddress/1 -> Relational1/2
  Data/1 -> Register1/1
  PortId/1 -> Relational1/1
  Write/1 -> Logical/2
  Register1/1 -> LatchedData/1

== system N3Z_tonetestprevious/User_Interface/OutputRegister/Subsystem7 ==
  Data : Inport
  PortId : Inport  Port=2
  Write : Inport  Port=3
  Logical : xbsIndex_r4/Logical  logical_function=AND  inputs=2  en=off  latency=0  precision=Full  arith_type=Unsigned  n_bits=8  bin_pt=2  align_bp=on  dbl_ovrd=off  block_type=logical
      settings: xl_area=[1 0 0 1 0 0 0]  block_version=VER_STRING_GOES_HERE
  PortAddress : xbsIndex_r4/Constant  const=2  gui_display_data_type=Fixed-point  arith_type=Unsigned  n_bits=8  bin_pt=0  preci_type=Single  exp_width=8  frac_width=24  explicit_period=on  period=fpgaclk  equ=P=C  opselect=C  inp2=PCIN>>17  opr=+  inp1=P  carry=CIN  dbl_ovrd=off  block_type=constant
      settings: block_version=VER_STRING_GOES_HERE
  Register1 : xbsIndex_r4/Register  init=hex2dec('5c')  rst=off  en=on  dbl_ovrd=off  block_type=register
      settings: xl_area=[4 8 0 0 0 0 0]  block_version=VER_STRING_GOES_HERE
  Relational1 : xbsIndex_r4/Relational  mode=a=b  op_type=Bool  en=off  latency=0  dbl_ovrd=off  block_type=relational
      settings: xl_area=[2 0 0 4 0 0 0]  block_version=VER_STRING_GOES_HERE
  LatchedData : Outport
  wires:
  Relational1/1 -> Logical/1
  Logical/1 -> Register1/2
  PortAddress/1 -> Relational1/2
  Data/1 -> Register1/1
  PortId/1 -> Relational1/1
  Write/1 -> Logical/2
  Register1/1 -> LatchedData/1

== system N3Z_tonetestprevious/User_Interface/OutputRegister/Subsystem8 ==
  Data : Inport
  PortId : Inport  Port=2
  Write : Inport  Port=3
  Logical : xbsIndex_r4/Logical  logical_function=AND  inputs=2  en=off  latency=0  precision=Full  arith_type=Unsigned  n_bits=8  bin_pt=2  align_bp=on  dbl_ovrd=off  block_type=logical
      settings: xl_area=[1 0 0 1 0 0 0]  block_version=VER_STRING_GOES_HERE
  PortAddress : xbsIndex_r4/Constant  const=8  gui_display_data_type=Fixed-point  arith_type=Unsigned  n_bits=8  bin_pt=0  preci_type=Single  exp_width=8  frac_width=24  explicit_period=on  period=fpgaclk  equ=P=C  opselect=C  inp2=PCIN>>17  opr=+  inp1=P  carry=CIN  dbl_ovrd=off  block_type=constant
      settings: block_version=VER_STRING_GOES_HERE
  Register1 : xbsIndex_r4/Register  init=0  rst=off  en=on  dbl_ovrd=off  block_type=register
      settings: xl_area=[4 8 0 0 0 0 0]  block_version=VER_STRING_GOES_HERE
  Relational1 : xbsIndex_r4/Relational  mode=a=b  op_type=Bool  en=off  latency=0  dbl_ovrd=off  block_type=relational
      settings: xl_area=[2 0 0 4 0 0 0]  block_version=VER_STRING_GOES_HERE
  LatchedData : Outport
  wires:
  Relational1/1 -> Logical/1
  Logical/1 -> Register1/2
  PortAddress/1 -> Relational1/2
  Data/1 -> Register1/1
  PortId/1 -> Relational1/1
  Write/1 -> Logical/2
  Register1/1 -> LatchedData/1

== system N3Z_tonetestprevious/User_Interface/OutputRegister/Subsystem9 ==
  Data : Inport
  PortId : Inport  Port=2
  Write : Inport  Port=3
  Logical : xbsIndex_r4/Logical  logical_function=AND  inputs=2  en=off  latency=0  precision=Full  arith_type=Unsigned  n_bits=8  bin_pt=2  align_bp=on  dbl_ovrd=off  block_type=logical
      settings: xl_area=[1 0 0 1 0 0 0]  block_version=VER_STRING_GOES_HERE
  PortAddress : xbsIndex_r4/Constant  const=9  gui_display_data_type=Fixed-point  arith_type=Unsigned  n_bits=8  bin_pt=0  preci_type=Single  exp_width=8  frac_width=24  explicit_period=on  period=fpgaclk  equ=P=C  opselect=C  inp2=PCIN>>17  opr=+  inp1=P  carry=CIN  dbl_ovrd=off  block_type=constant
      settings: block_version=VER_STRING_GOES_HERE
  Register1 : xbsIndex_r4/Register  init=0  rst=off  en=on  dbl_ovrd=off  block_type=register
      settings: xl_area=[4 8 0 0 0 0 0]  block_version=VER_STRING_GOES_HERE
  Relational1 : xbsIndex_r4/Relational  mode=a=b  op_type=Bool  en=off  latency=0  dbl_ovrd=off  block_type=relational
      settings: xl_area=[2 0 0 4 0 0 0]  block_version=VER_STRING_GOES_HERE
  LatchedData : Outport
  wires:
  Relational1/1 -> Logical/1
  Logical/1 -> Register1/2
  PortAddress/1 -> Relational1/2
  Data/1 -> Register1/1
  PortId/1 -> Relational1/1
  Write/1 -> Logical/2
  Register1/1 -> LatchedData/1

== system N3Z_tonetestprevious/DemodulationSSB1/FilterStreamIntegration/TrigDistrib/3LineTo8Way ==
  In1 : Inport
  BitBasher : xbsIndex_r4/BitBasher  bitexpr=|  display_expr=off  sr_1=1  arith_type1=Unsigned  bin_pt1=0  sr_2=2  arith_type2=Unsigned  bin_pt2=0  sr_3=3  arith_type3=Unsigned  bin_pt3=0  sr_4=4  arith_type4=Unsigned  bin_pt4=0  dbl_ovrd=off  block_type=bitbasher
      | <html><head><meta name="qrichtext" content="1" /></head><body style="font-size:8pt;font-family:MS Shell Dlg">
      | <p>B0={a[0]}<br />B1={a[1]}<br />B2={a[2]}<br /></p>
      | </body></html>
      settings: block_version=8.2.02
      settings: infoedit=|
      | Allows
      |      extraction, concatenation and augmentation of bits
  BitBasher1 : xbsIndex_r4/BitBasher  bitexpr=|  display_expr=off  sr_1=1  arith_type1=Unsigned  bin_pt1=0  sr_2=2  arith_type2=Unsigned  bin_pt2=0  sr_3=3  arith_type3=Unsigned  bin_pt3=0  sr_4=4  arith_type4=Unsigned  bin_pt4=0  dbl_ovrd=off  block_type=bitbasher
      | <html><head><meta name="qrichtext" content="1" /></head><body style="font-size:8pt;font-family:MS Shell Dlg">
      | <p>B3={a[3]}<br />B4={a[4]}<br />B5={a[5]}<br /></p>
      | </body></html>
      settings: block_version=8.2.02
      settings: infoedit=|
      | Allows
      |      extraction, concatenation and augmentation of bits
  BitBasher2 : xbsIndex_r4/BitBasher  bitexpr=|  display_expr=off  sr_1=1  arith_type1=Unsigned  bin_pt1=0  sr_2=2  arith_type2=Unsigned  bin_pt2=0  sr_3=3  arith_type3=Unsigned  bin_pt3=0  sr_4=4  arith_type4=Unsigned  bin_pt4=0  dbl_ovrd=off  block_type=bitbasher
      | <html><head><meta name="qrichtext" content="1" /></head><body style="font-size:8pt;font-family:MS Shell Dlg">
      | <p>B6={a[6]}<br />B7={a[7]}<br /><br /></p>
      | </body></html>
      settings: block_version=8.2.02
      settings: infoedit=|
      | Allows
      |      extraction, concatenation and augmentation of bits
  Convert{,1..7} (8 alike) : xbsIndex_r4/Convert  gui_display_data_type=Fixed-point  arith_type=Boolean  n_bits=16  bin_pt=14  float_type=Single  exp_bits=8  fraction_bits=24  quantization=Truncate  overflow=Wrap  en=off  latency=0  pipeline=off  dbl_ovrd=off  block_type=convert
      settings: xl_area=[0 0 0 0 0 0 0]  block_version=8.2.02
  ROM : xbsIndex_r4/ROM  depth=8  initVector=2.^[0:7]  distributed_mem=Distributed memory  rst=off  init_reg=0  en=off  latency=1  gui_display_data_type=Fixed-point  arith_type=Unsigned  n_bits=8  bin_pt=0  preci_type=Single  exp_width=8  frac_width=24  optimize=Area  use_rpm=on  dbl_ovrd=off  block_type=sprom
      settings: xl_area=[4 8 0 8 0 0 0]  block_version=8.2.02
  Out1 : Outport
  Out2 : Outport  Port=2
  Out3 : Outport  Port=3
  Out4 : Outport  Port=4
  Out5 : Outport  Port=5
  Out6 : Outport  Port=6
  Out7 : Outport  Port=7
  Out8 : Outport  Port=8
  wires:
  ROM/1 -> BitBasher/1, BitBasher1/1, BitBasher2/1
  BitBasher/1 -> Convert/1
  BitBasher/2 -> Convert1/1
  In1/1 -> ROM/1
  BitBasher/3 -> Convert2/1
  BitBasher1/1 -> Convert3/1
  BitBasher1/2 -> Convert4/1
  BitBasher1/3 -> Convert5/1
  BitBasher2/1 -> Convert6/1
  BitBasher2/2 -> Convert7/1
  Convert/1 -> Out1/1
  Convert1/1 -> Out2/1
  Convert2/1 -> Out3/1
  Convert3/1 -> Out4/1
  Convert4/1 -> Out5/1
  Convert5/1 -> Out6/1
  Convert6/1 -> Out7/1
  Convert7/1 -> Out8/1
